simulink model "TST_CoVMD_TrqLeadCoord"  (R2016b)
settings: Solver=FixedStepDiscrete  StartTime=0.0  StopTime=simTime  FixedStep=sampleTime  RelTol=1e-3
values from neighbouring files (symbols this model uses):
  testCase = 1    [initTST_CoVMD_TrqLeadCoord_001.m]    (also in initTST_CoVMD_TrqLeadCoord_002.m = 2; initTST_CoVMD_TrqLeadCoord_003.m = 3)
libraries: simulink x16, UnitTest_Lib x12
settings Model: Creator=zhengjinyan  LastModifiedBy=zhengjinyan
settings DebuggingCC: SignalRangeChecking=error

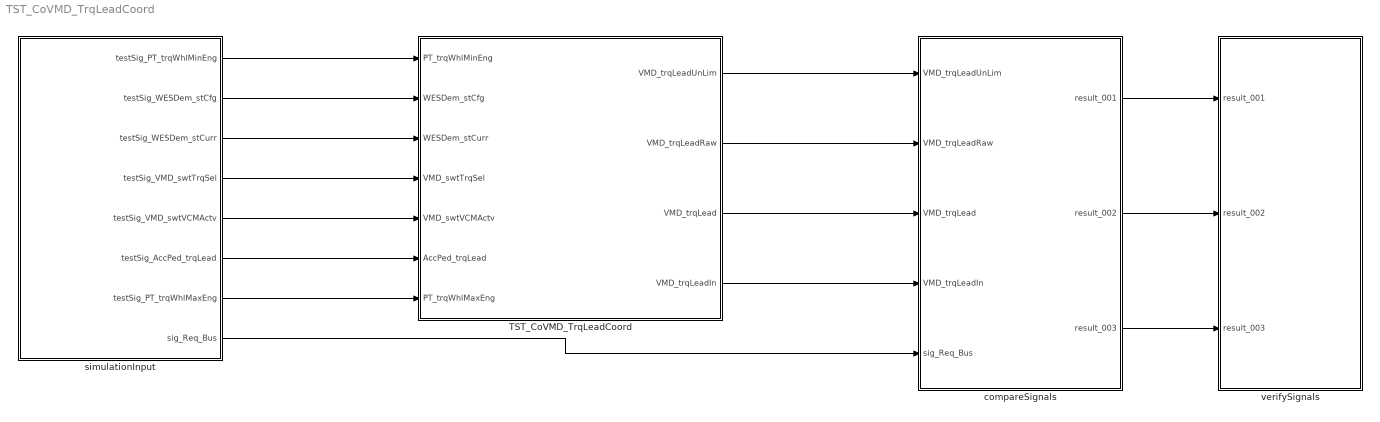
== system TST_CoVMD_TrqLeadCoord ==
  TST_CoVMD_TrqLeadCoord : Subsystem
  compareSignals : Subsystem
  simulationInput : Subsystem
  verifySignals : Subsystem
  wires:
  simulationInput/1(testSig_PT_trqWhlMinEng) -> TST_CoVMD_TrqLeadCoord/1(PT_trqWhlMinEng)
  simulationInput/2(testSig_WESDem_stCfg) -> TST_CoVMD_TrqLeadCoord/2(WESDem_stCfg)
  simulationInput/3(testSig_WESDem_stCurr) -> TST_CoVMD_TrqLeadCoord/3(WESDem_stCurr)
  simulationInput/4(testSig_VMD_swtTrqSel) -> TST_CoVMD_TrqLeadCoord/4(VMD_swtTrqSel)
  simulationInput/5(testSig_VMD_swtVCMActv) -> TST_CoVMD_TrqLeadCoord/5(VMD_swtVCMActv)
  simulationInput/6(testSig_AccPed_trqLead) -> TST_CoVMD_TrqLeadCoord/6(AccPed_trqLead)
  simulationInput/7(testSig_PT_trqWhlMaxEng) -> TST_CoVMD_TrqLeadCoord/7(PT_trqWhlMaxEng)
  TST_CoVMD_TrqLeadCoord/1(VMD_trqLeadUnLim) -> compareSignals/1(VMD_trqLeadUnLim)
  TST_CoVMD_TrqLeadCoord/2(VMD_trqLeadRaw) -> compareSignals/2(VMD_trqLeadRaw)
  TST_CoVMD_TrqLeadCoord/3(VMD_trqLead) -> compareSignals/3(VMD_trqLead)
  TST_CoVMD_TrqLeadCoord/4(VMD_trqLeadIn) -> compareSignals/4(VMD_trqLeadIn)
  simulationInput/8(sig_Req_Bus) -> compareSignals/5(sig_Req_Bus)
  compareSignals/1(result_001) -> verifySignals/1(result_001)
  compareSignals/2(result_002) -> verifySignals/2(result_002)
  compareSignals/3(result_003) -> verifySignals/3(result_003)

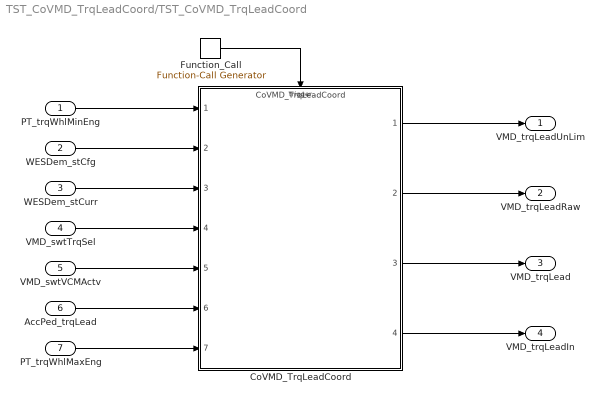
== system TST_CoVMD_TrqLeadCoord/TST_CoVMD_TrqLeadCoord ==
  PT_trqWhlMinEng : Inport
  WESDem_stCfg : Inport  Port=2
  WESDem_stCurr : Inport  Port=3
  VMD_swtTrqSel : Inport  Port=4
  VMD_swtVCMActv : Inport  Port=5
  AccPed_trqLead : Inport  Port=6
  PT_trqWhlMaxEng : Inport  Port=7
  CoVMD_TrqLeadCoord : ModelReference  ModelNameDialog=CoVMD_TrqLeadCoord  SimulationMode=Normal  ModelReferenceVersion=1.13  TriggerPortName=function  TriggerPortTriggerType=function-call  TriggerPortStatesWhenEnabling=held
  Function_Call : simulink/Ports & Subsystems/Function-Call Generator  sample_time=sampleTime  numberOfIterations=1
  VMD_trqLeadUnLim : Outport
  VMD_trqLeadRaw : Outport  Port=2
  VMD_trqLead : Outport  Port=3
  VMD_trqLeadIn : Outport  Port=4
  wires:
  Function_Call/1 -> CoVMD_TrqLeadCoord/Trigger
  PT_trqWhlMinEng/1 -> CoVMD_TrqLeadCoord/1
  WESDem_stCfg/1 -> CoVMD_TrqLeadCoord/2
  WESDem_stCurr/1 -> CoVMD_TrqLeadCoord/3
  VMD_swtTrqSel/1 -> CoVMD_TrqLeadCoord/4
  VMD_swtVCMActv/1 -> CoVMD_TrqLeadCoord/5
  AccPed_trqLead/1 -> CoVMD_TrqLeadCoord/6
  PT_trqWhlMaxEng/1 -> CoVMD_TrqLeadCoord/7
  CoVMD_TrqLeadCoord/1 -> VMD_trqLeadUnLim/1
  CoVMD_TrqLeadCoord/2 -> VMD_trqLeadRaw/1
  CoVMD_TrqLeadCoord/3 -> VMD_trqLead/1
  CoVMD_TrqLeadCoord/4 -> VMD_trqLeadIn/1

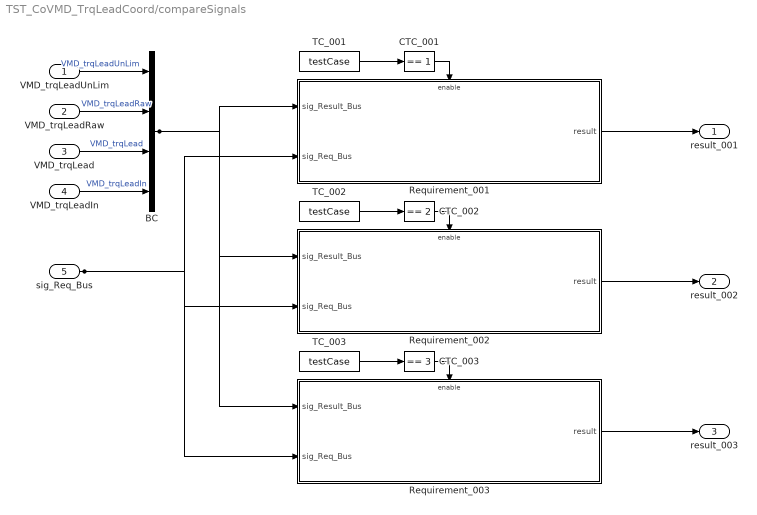
== system TST_CoVMD_TrqLeadCoord/compareSignals ==
  VMD_trqLeadUnLim : Inport
  VMD_trqLeadRaw : Inport  Port=2
  VMD_trqLead : Inport  Port=3
  VMD_trqLeadIn : Inport  Port=4
  sig_Req_Bus : Inport  Port=5
  BC : BusCreator  Inputs=4
  CTC_001 : simulink/Logic and Bit Operations/Compare To Constant  relop===  const=1  OutDataTypeStr=boolean
  CTC_002 : simulink/Logic and Bit Operations/Compare To Constant  relop===  const=2  OutDataTypeStr=boolean
  CTC_003 : simulink/Logic and Bit Operations/Compare To Constant  relop===  const=3  OutDataTypeStr=boolean
  Requirement_001 : Subsystem
  Requirement_002 : Subsystem
  Requirement_003 : Subsystem
  TC_001 : Constant  Value=testCase
  TC_002 : Constant  Value=testCase
  TC_003 : Constant  Value=testCase
  result_001 : Outport
  result_002 : Outport  Port=2
  result_003 : Outport  Port=3
  wires:
  VMD_trqLeadUnLim/1 -> BC/1  "VMD_trqLeadUnLim"
  VMD_trqLeadRaw/1 -> BC/2  "VMD_trqLeadRaw"
  VMD_trqLead/1 -> BC/3  "VMD_trqLead"
  VMD_trqLeadIn/1 -> BC/4  "VMD_trqLeadIn"
  TC_001/1 -> CTC_001/1
  CTC_001/1 -> Requirement_001/Enable
  sig_Req_Bus/1 -> Requirement_001/2(sig_Req_Bus), Requirement_002/2(sig_Req_Bus), Requirement_003/2(sig_Req_Bus)
  BC/1 -> Requirement_001/1(sig_Result_Bus), Requirement_002/1(sig_Result_Bus), Requirement_003/1(sig_Result_Bus)
  Requirement_001/1(result) -> result_001/1
  TC_002/1 -> CTC_002/1
  CTC_002/1 -> Requirement_002/Enable
  Requirement_002/1(result) -> result_002/1
  TC_003/1 -> CTC_003/1
  CTC_003/1 -> Requirement_003/Enable
  Requirement_003/1(result) -> result_003/1

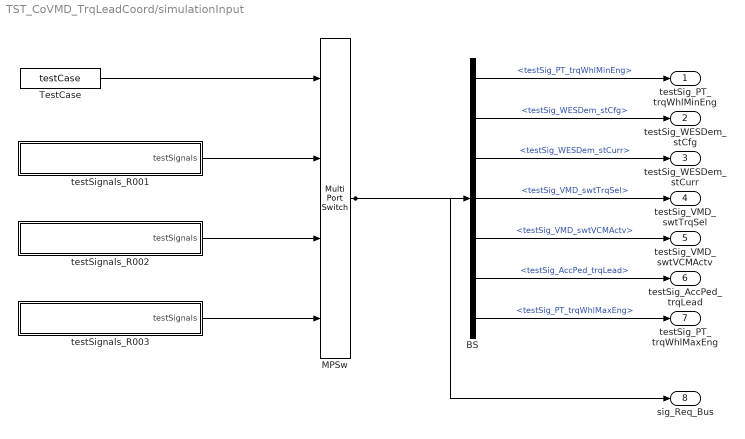
== system TST_CoVMD_TrqLeadCoord/simulationInput ==
  BS : BusSelector  OutputSignals=testSig_PT_trqWhlMinEng,testSig_WESDem_stCfg,testSig_WESDem_stCurr,testSig_VMD_swtTrqSel,testSig_VMD_swtVCMActv,testSig_AccPed_trqLead,testSig_PT_trqWhlMaxEng
  MPSw : MultiPortSwitch  SaturateOnIntegerOverflow=on  InputSameDT=on
  TestCase : Constant  Value=testCase
  testSignals_R001 : Subsystem
  testSignals_R002 : Subsystem
  testSignals_R003 : Subsystem
  testSig_PT_trqWhlMinEng : Outport
  testSig_WESDem_stCfg : Outport  Port=2
  testSig_WESDem_stCurr : Outport  Port=3
  testSig_VMD_swtTrqSel : Outport  Port=4
  testSig_VMD_swtVCMActv : Outport  Port=5
  testSig_AccPed_trqLead : Outport  Port=6
  testSig_PT_trqWhlMaxEng : Outport  Port=7
  sig_Req_Bus : Outport  Port=8
  wires:
  BS/1 -> testSig_PT_trqWhlMinEng/1  "<testSig_PT_trqWhlMinEng>"
  BS/2 -> testSig_WESDem_stCfg/1  "<testSig_WESDem_stCfg>"
  BS/3 -> testSig_WESDem_stCurr/1  "<testSig_WESDem_stCurr>"
  BS/4 -> testSig_VMD_swtTrqSel/1  "<testSig_VMD_swtTrqSel>"
  BS/5 -> testSig_VMD_swtVCMActv/1  "<testSig_VMD_swtVCMActv>"
  BS/6 -> testSig_AccPed_trqLead/1  "<testSig_AccPed_trqLead>"
  BS/7 -> testSig_PT_trqWhlMaxEng/1  "<testSig_PT_trqWhlMaxEng>"
  MPSw/1 -> BS/1, sig_Req_Bus/1
  TestCase/1 -> MPSw/1
  testSignals_R001/1(testSignals) -> MPSw/2
  testSignals_R002/1(testSignals) -> MPSw/3
  testSignals_R003/1(testSignals) -> MPSw/4

== system TST_CoVMD_TrqLeadCoord/verifySignals ==
  result_001 : Inport
  result_002 : Inport  Port=2
  result_003 : Inport  Port=3
  Assertion_001 : Assertion  Enabled=off
  Assertion_002 : Assertion  Enabled=off
  Assertion_003 : Assertion  Enabled=off
  wires:
  result_001/1 -> Assertion_001/1
  result_002/1 -> Assertion_002/1
  result_003/1 -> Assertion_003/1

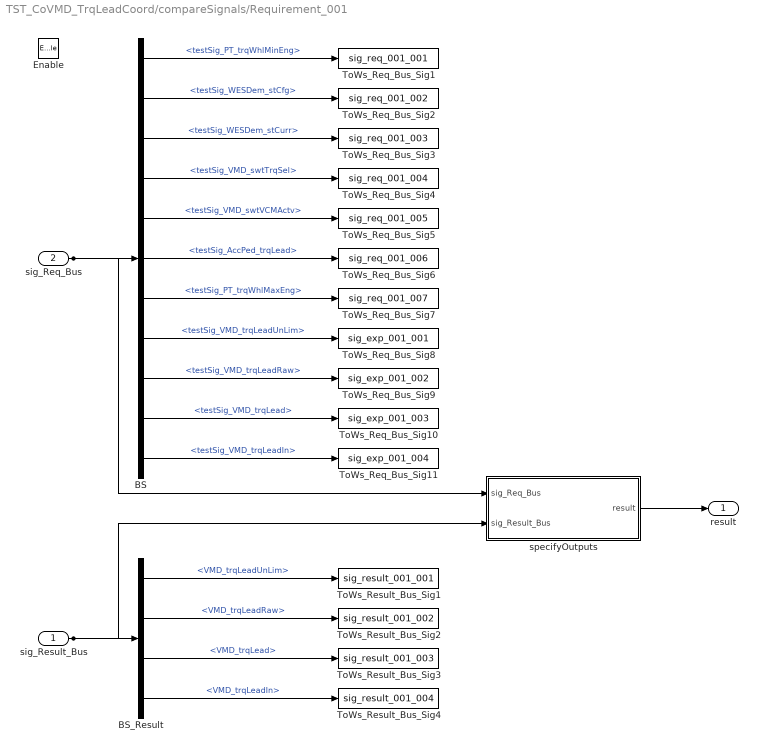
== system TST_CoVMD_TrqLeadCoord/compareSignals/Requirement_001 ==
  sig_Result_Bus : Inport
  sig_Req_Bus : Inport  Port=2
  Enable : EnablePort
  BS : BusSelector  OutputSignals=testSig_PT_trqWhlMinEng,testSig_WESDem_stCfg,testSig_WESDem_stCurr,testSig_VMD_swtTrqSel,testSig_VMD_swtVCMActv,testSig_AccPed_trqLead,testSig_PT_trqWhlMaxEng,testSig_VMD_trqLeadUnLim,testSig_VMD_trqLeadRaw,testSig_VMD_trqLead,testSig_VMD_trqLeadIn
  BS_Result : BusSelector  OutputSignals=VMD_trqLeadUnLim,VMD_trqLeadRaw,VMD_trqLead,VMD_trqLeadIn
  ToWs_Req_Bus_Sig1 : ToWorkspace  VariableName=sig_req_001_001  SaveFormat=Structure With Time
  ToWs_Req_Bus_Sig10 : ToWorkspace  VariableName=sig_exp_001_003  SaveFormat=Structure With Time
  ToWs_Req_Bus_Sig11 : ToWorkspace  VariableName=sig_exp_001_004  SaveFormat=Structure With Time
  ToWs_Req_Bus_Sig2 : ToWorkspace  VariableName=sig_req_001_002  SaveFormat=Structure With Time
  ToWs_Req_Bus_Sig3 : ToWorkspace  VariableName=sig_req_001_003  SaveFormat=Structure With Time
  ToWs_Req_Bus_Sig4 : ToWorkspace  VariableName=sig_req_001_004  SaveFormat=Structure With Time
  ToWs_Req_Bus_Sig5 : ToWorkspace  VariableName=sig_req_001_005  SaveFormat=Structure With Time
  ToWs_Req_Bus_Sig6 : ToWorkspace  VariableName=sig_req_001_006  SaveFormat=Structure With Time
  ToWs_Req_Bus_Sig7 : ToWorkspace  VariableName=sig_req_001_007  SaveFormat=Structure With Time
  ToWs_Req_Bus_Sig8 : ToWorkspace  VariableName=sig_exp_001_001  SaveFormat=Structure With Time
  ToWs_Req_Bus_Sig9 : ToWorkspace  VariableName=sig_exp_001_002  SaveFormat=Structure With Time
  ToWs_Result_Bus_Sig1 : ToWorkspace  VariableName=sig_result_001_001  SaveFormat=Structure With Time
  ToWs_Result_Bus_Sig2 : ToWorkspace  VariableName=sig_result_001_002  SaveFormat=Structure With Time
  ToWs_Result_Bus_Sig3 : ToWorkspace  VariableName=sig_result_001_003  SaveFormat=Structure With Time
  ToWs_Result_Bus_Sig4 : ToWorkspace  VariableName=sig_result_001_004  SaveFormat=Structure With Time
  specifyOutputs : Subsystem
  result : Outport
  wires:
  sig_Req_Bus/1 -> BS/1, specifyOutputs/1(sig_Req_Bus)
  BS/1 -> ToWs_Req_Bus_Sig1/1  "<testSig_PT_trqWhlMinEng>"
  BS/2 -> ToWs_Req_Bus_Sig2/1  "<testSig_WESDem_stCfg>"
  BS/3 -> ToWs_Req_Bus_Sig3/1  "<testSig_WESDem_stCurr>"
  BS/4 -> ToWs_Req_Bus_Sig4/1  "<testSig_VMD_swtTrqSel>"
  BS/5 -> ToWs_Req_Bus_Sig5/1  "<testSig_VMD_swtVCMActv>"
  BS/6 -> ToWs_Req_Bus_Sig6/1  "<testSig_AccPed_trqLead>"
  BS/7 -> ToWs_Req_Bus_Sig7/1  "<testSig_PT_trqWhlMaxEng>"
  BS/8 -> ToWs_Req_Bus_Sig8/1  "<testSig_VMD_trqLeadUnLim>"
  BS/9 -> ToWs_Req_Bus_Sig9/1  "<testSig_VMD_trqLeadRaw>"
  BS/10 -> ToWs_Req_Bus_Sig10/1  "<testSig_VMD_trqLead>"
  BS/11 -> ToWs_Req_Bus_Sig11/1  "<testSig_VMD_trqLeadIn>"
  sig_Result_Bus/1 -> BS_Result/1, specifyOutputs/2(sig_Result_Bus)
  BS_Result/1 -> ToWs_Result_Bus_Sig1/1  "<VMD_trqLeadUnLim>"
  BS_Result/2 -> ToWs_Result_Bus_Sig2/1  "<VMD_trqLeadRaw>"
  BS_Result/3 -> ToWs_Result_Bus_Sig3/1  "<VMD_trqLead>"
  BS_Result/4 -> ToWs_Result_Bus_Sig4/1  "<VMD_trqLeadIn>"
  specifyOutputs/1(result) -> result/1

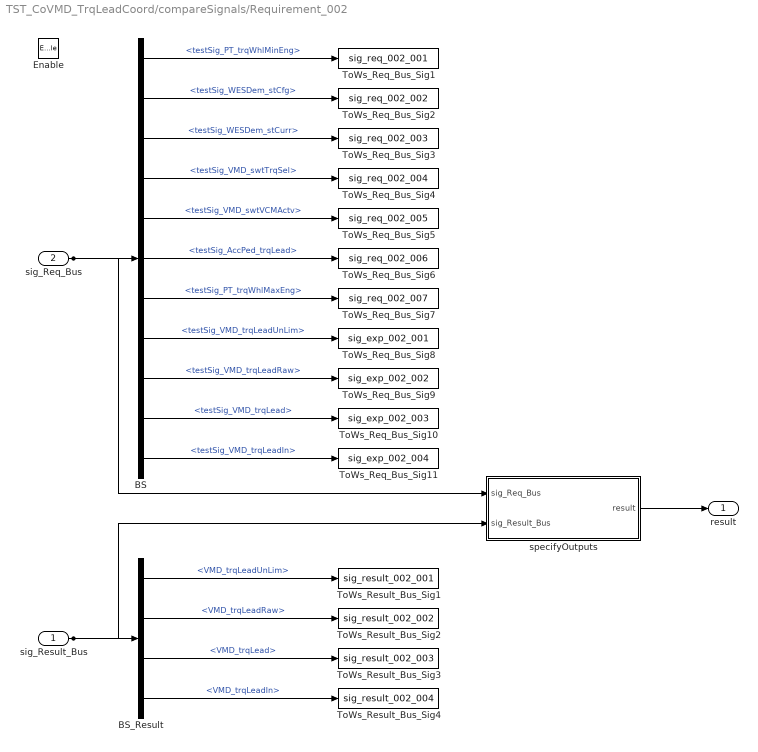
== system TST_CoVMD_TrqLeadCoord/compareSignals/Requirement_002 ==
  sig_Result_Bus : Inport
  sig_Req_Bus : Inport  Port=2
  Enable : EnablePort
  BS : BusSelector  OutputSignals=testSig_PT_trqWhlMinEng,testSig_WESDem_stCfg,testSig_WESDem_stCurr,testSig_VMD_swtTrqSel,testSig_VMD_swtVCMActv,testSig_AccPed_trqLead,testSig_PT_trqWhlMaxEng,testSig_VMD_trqLeadUnLim,testSig_VMD_trqLeadRaw,testSig_VMD_trqLead,testSig_VMD_trqLeadIn
  BS_Result : BusSelector  OutputSignals=VMD_trqLeadUnLim,VMD_trqLeadRaw,VMD_trqLead,VMD_trqLeadIn
  ToWs_Req_Bus_Sig1 : ToWorkspace  VariableName=sig_req_002_001  SaveFormat=Structure With Time
  ToWs_Req_Bus_Sig10 : ToWorkspace  VariableName=sig_exp_002_003  SaveFormat=Structure With Time
  ToWs_Req_Bus_Sig11 : ToWorkspace  VariableName=sig_exp_002_004  SaveFormat=Structure With Time
  ToWs_Req_Bus_Sig2 : ToWorkspace  VariableName=sig_req_002_002  SaveFormat=Structure With Time
  ToWs_Req_Bus_Sig3 : ToWorkspace  VariableName=sig_req_002_003  SaveFormat=Structure With Time
  ToWs_Req_Bus_Sig4 : ToWorkspace  VariableName=sig_req_002_004  SaveFormat=Structure With Time
  ToWs_Req_Bus_Sig5 : ToWorkspace  VariableName=sig_req_002_005  SaveFormat=Structure With Time
  ToWs_Req_Bus_Sig6 : ToWorkspace  VariableName=sig_req_002_006  SaveFormat=Structure With Time
  ToWs_Req_Bus_Sig7 : ToWorkspace  VariableName=sig_req_002_007  SaveFormat=Structure With Time
  ToWs_Req_Bus_Sig8 : ToWorkspace  VariableName=sig_exp_002_001  SaveFormat=Structure With Time
  ToWs_Req_Bus_Sig9 : ToWorkspace  VariableName=sig_exp_002_002  SaveFormat=Structure With Time
  ToWs_Result_Bus_Sig1 : ToWorkspace  VariableName=sig_result_002_001  SaveFormat=Structure With Time
  ToWs_Result_Bus_Sig2 : ToWorkspace  VariableName=sig_result_002_002  SaveFormat=Structure With Time
  ToWs_Result_Bus_Sig3 : ToWorkspace  VariableName=sig_result_002_003  SaveFormat=Structure With Time
  ToWs_Result_Bus_Sig4 : ToWorkspace  VariableName=sig_result_002_004  SaveFormat=Structure With Time
  specifyOutputs : Subsystem
  result : Outport
  wires:
  sig_Req_Bus/1 -> BS/1, specifyOutputs/1(sig_Req_Bus)
  BS/1 -> ToWs_Req_Bus_Sig1/1  "<testSig_PT_trqWhlMinEng>"
  BS/2 -> ToWs_Req_Bus_Sig2/1  "<testSig_WESDem_stCfg>"
  BS/3 -> ToWs_Req_Bus_Sig3/1  "<testSig_WESDem_stCurr>"
  BS/4 -> ToWs_Req_Bus_Sig4/1  "<testSig_VMD_swtTrqSel>"
  BS/5 -> ToWs_Req_Bus_Sig5/1  "<testSig_VMD_swtVCMActv>"
  BS/6 -> ToWs_Req_Bus_Sig6/1  "<testSig_AccPed_trqLead>"
  BS/7 -> ToWs_Req_Bus_Sig7/1  "<testSig_PT_trqWhlMaxEng>"
  BS/8 -> ToWs_Req_Bus_Sig8/1  "<testSig_VMD_trqLeadUnLim>"
  BS/9 -> ToWs_Req_Bus_Sig9/1  "<testSig_VMD_trqLeadRaw>"
  BS/10 -> ToWs_Req_Bus_Sig10/1  "<testSig_VMD_trqLead>"
  BS/11 -> ToWs_Req_Bus_Sig11/1  "<testSig_VMD_trqLeadIn>"
  sig_Result_Bus/1 -> BS_Result/1, specifyOutputs/2(sig_Result_Bus)
  BS_Result/1 -> ToWs_Result_Bus_Sig1/1  "<VMD_trqLeadUnLim>"
  BS_Result/2 -> ToWs_Result_Bus_Sig2/1  "<VMD_trqLeadRaw>"
  BS_Result/3 -> ToWs_Result_Bus_Sig3/1  "<VMD_trqLead>"
  BS_Result/4 -> ToWs_Result_Bus_Sig4/1  "<VMD_trqLeadIn>"
  specifyOutputs/1(result) -> result/1

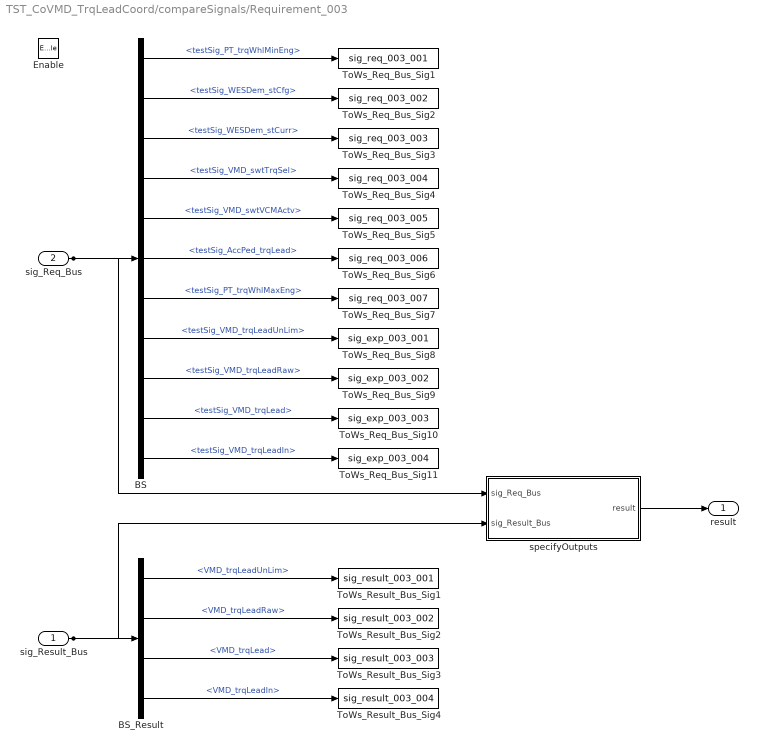
== system TST_CoVMD_TrqLeadCoord/compareSignals/Requirement_003 ==
  sig_Result_Bus : Inport
  sig_Req_Bus : Inport  Port=2
  Enable : EnablePort
  BS : BusSelector  OutputSignals=testSig_PT_trqWhlMinEng,testSig_WESDem_stCfg,testSig_WESDem_stCurr,testSig_VMD_swtTrqSel,testSig_VMD_swtVCMActv,testSig_AccPed_trqLead,testSig_PT_trqWhlMaxEng,testSig_VMD_trqLeadUnLim,testSig_VMD_trqLeadRaw,testSig_VMD_trqLead,testSig_VMD_trqLeadIn
  BS_Result : BusSelector  OutputSignals=VMD_trqLeadUnLim,VMD_trqLeadRaw,VMD_trqLead,VMD_trqLeadIn
  ToWs_Req_Bus_Sig1 : ToWorkspace  VariableName=sig_req_003_001  SaveFormat=Structure With Time
  ToWs_Req_Bus_Sig10 : ToWorkspace  VariableName=sig_exp_003_003  SaveFormat=Structure With Time
  ToWs_Req_Bus_Sig11 : ToWorkspace  VariableName=sig_exp_003_004  SaveFormat=Structure With Time
  ToWs_Req_Bus_Sig2 : ToWorkspace  VariableName=sig_req_003_002  SaveFormat=Structure With Time
  ToWs_Req_Bus_Sig3 : ToWorkspace  VariableName=sig_req_003_003  SaveFormat=Structure With Time
  ToWs_Req_Bus_Sig4 : ToWorkspace  VariableName=sig_req_003_004  SaveFormat=Structure With Time
  ToWs_Req_Bus_Sig5 : ToWorkspace  VariableName=sig_req_003_005  SaveFormat=Structure With Time
  ToWs_Req_Bus_Sig6 : ToWorkspace  VariableName=sig_req_003_006  SaveFormat=Structure With Time
  ToWs_Req_Bus_Sig7 : ToWorkspace  VariableName=sig_req_003_007  SaveFormat=Structure With Time
  ToWs_Req_Bus_Sig8 : ToWorkspace  VariableName=sig_exp_003_001  SaveFormat=Structure With Time
  ToWs_Req_Bus_Sig9 : ToWorkspace  VariableName=sig_exp_003_002  SaveFormat=Structure With Time
  ToWs_Result_Bus_Sig1 : ToWorkspace  VariableName=sig_result_003_001  SaveFormat=Structure With Time
  ToWs_Result_Bus_Sig2 : ToWorkspace  VariableName=sig_result_003_002  SaveFormat=Structure With Time
  ToWs_Result_Bus_Sig3 : ToWorkspace  VariableName=sig_result_003_003  SaveFormat=Structure With Time
  ToWs_Result_Bus_Sig4 : ToWorkspace  VariableName=sig_result_003_004  SaveFormat=Structure With Time
  specifyOutputs : Subsystem
  result : Outport
  wires:
  sig_Req_Bus/1 -> BS/1, specifyOutputs/1(sig_Req_Bus)
  BS/1 -> ToWs_Req_Bus_Sig1/1  "<testSig_PT_trqWhlMinEng>"
  BS/2 -> ToWs_Req_Bus_Sig2/1  "<testSig_WESDem_stCfg>"
  BS/3 -> ToWs_Req_Bus_Sig3/1  "<testSig_WESDem_stCurr>"
  BS/4 -> ToWs_Req_Bus_Sig4/1  "<testSig_VMD_swtTrqSel>"
  BS/5 -> ToWs_Req_Bus_Sig5/1  "<testSig_VMD_swtVCMActv>"
  BS/6 -> ToWs_Req_Bus_Sig6/1  "<testSig_AccPed_trqLead>"
  BS/7 -> ToWs_Req_Bus_Sig7/1  "<testSig_PT_trqWhlMaxEng>"
  BS/8 -> ToWs_Req_Bus_Sig8/1  "<testSig_VMD_trqLeadUnLim>"
  BS/9 -> ToWs_Req_Bus_Sig9/1  "<testSig_VMD_trqLeadRaw>"
  BS/10 -> ToWs_Req_Bus_Sig10/1  "<testSig_VMD_trqLead>"
  BS/11 -> ToWs_Req_Bus_Sig11/1  "<testSig_VMD_trqLeadIn>"
  sig_Result_Bus/1 -> BS_Result/1, specifyOutputs/2(sig_Result_Bus)
  BS_Result/1 -> ToWs_Result_Bus_Sig1/1  "<VMD_trqLeadUnLim>"
  BS_Result/2 -> ToWs_Result_Bus_Sig2/1  "<VMD_trqLeadRaw>"
  BS_Result/3 -> ToWs_Result_Bus_Sig3/1  "<VMD_trqLead>"
  BS_Result/4 -> ToWs_Result_Bus_Sig4/1  "<VMD_trqLeadIn>"
  specifyOutputs/1(result) -> result/1

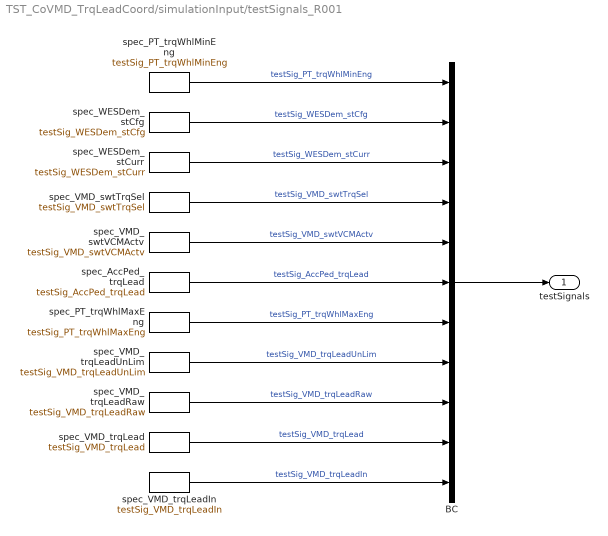
== system TST_CoVMD_TrqLeadCoord/simulationInput/testSignals_R001 ==
  BC : BusCreator  Inputs=11
  spec_AccPed_trqLead : FromWorkspace  VariableName=testSig_AccPed_trqLead  Interpolate=off  OutputAfterFinalValue=Holding final value
  spec_PT_trqWhlMaxEng : FromWorkspace  VariableName=testSig_PT_trqWhlMaxEng  Interpolate=off  OutputAfterFinalValue=Holding final value
  spec_PT_trqWhlMinEng : FromWorkspace  VariableName=testSig_PT_trqWhlMinEng  Interpolate=off  OutputAfterFinalValue=Holding final value
  spec_VMD_swtTrqSel : FromWorkspace  VariableName=testSig_VMD_swtTrqSel  Interpolate=off  OutputAfterFinalValue=Holding final value
  spec_VMD_swtVCMActv : FromWorkspace  VariableName=testSig_VMD_swtVCMActv  Interpolate=off  OutputAfterFinalValue=Holding final value
  spec_VMD_trqLead : FromWorkspace  VariableName=testSig_VMD_trqLead  Interpolate=off  OutputAfterFinalValue=Holding final value
  spec_VMD_trqLeadIn : FromWorkspace  VariableName=testSig_VMD_trqLeadIn  Interpolate=off  OutputAfterFinalValue=Holding final value
  spec_VMD_trqLeadRaw : FromWorkspace  VariableName=testSig_VMD_trqLeadRaw  Interpolate=off  OutputAfterFinalValue=Holding final value
  spec_VMD_trqLeadUnLim : FromWorkspace  VariableName=testSig_VMD_trqLeadUnLim  Interpolate=off  OutputAfterFinalValue=Holding final value
  spec_WESDem_stCfg : FromWorkspace  VariableName=testSig_WESDem_stCfg  Interpolate=off  OutputAfterFinalValue=Holding final value
  spec_WESDem_stCurr : FromWorkspace  VariableName=testSig_WESDem_stCurr  Interpolate=off  OutputAfterFinalValue=Holding final value
  testSignals : Outport
  wires:
  BC/1 -> testSignals/1
  spec_PT_trqWhlMinEng/1 -> BC/1  "testSig_PT_trqWhlMinEng"
  spec_WESDem_stCfg/1 -> BC/2  "testSig_WESDem_stCfg"
  spec_WESDem_stCurr/1 -> BC/3  "testSig_WESDem_stCurr"
  spec_VMD_swtTrqSel/1 -> BC/4  "testSig_VMD_swtTrqSel"
  spec_VMD_swtVCMActv/1 -> BC/5  "testSig_VMD_swtVCMActv"
  spec_AccPed_trqLead/1 -> BC/6  "testSig_AccPed_trqLead"
  spec_PT_trqWhlMaxEng/1 -> BC/7  "testSig_PT_trqWhlMaxEng"
  spec_VMD_trqLeadUnLim/1 -> BC/8  "testSig_VMD_trqLeadUnLim"
  spec_VMD_trqLeadRaw/1 -> BC/9  "testSig_VMD_trqLeadRaw"
  spec_VMD_trqLead/1 -> BC/10  "testSig_VMD_trqLead"
  spec_VMD_trqLeadIn/1 -> BC/11  "testSig_VMD_trqLeadIn"

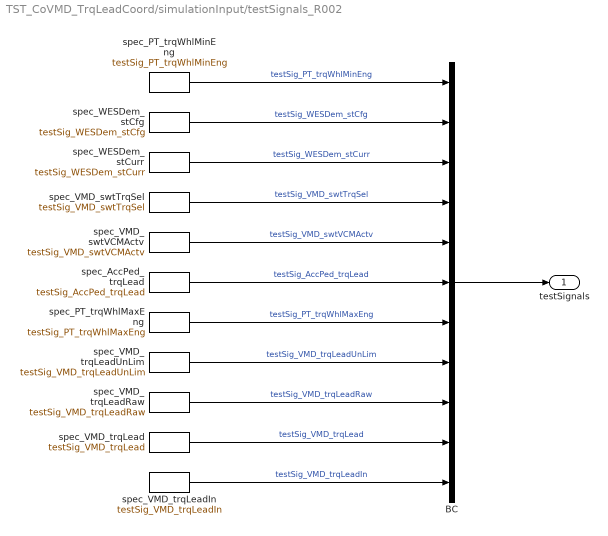
== system TST_CoVMD_TrqLeadCoord/simulationInput/testSignals_R002 ==
  BC : BusCreator  Inputs=11
  spec_AccPed_trqLead : FromWorkspace  VariableName=testSig_AccPed_trqLead  Interpolate=off  OutputAfterFinalValue=Holding final value
  spec_PT_trqWhlMaxEng : FromWorkspace  VariableName=testSig_PT_trqWhlMaxEng  Interpolate=off  OutputAfterFinalValue=Holding final value
  spec_PT_trqWhlMinEng : FromWorkspace  VariableName=testSig_PT_trqWhlMinEng  Interpolate=off  OutputAfterFinalValue=Holding final value
  spec_VMD_swtTrqSel : FromWorkspace  VariableName=testSig_VMD_swtTrqSel  Interpolate=off  OutputAfterFinalValue=Holding final value
  spec_VMD_swtVCMActv : FromWorkspace  VariableName=testSig_VMD_swtVCMActv  Interpolate=off  OutputAfterFinalValue=Holding final value
  spec_VMD_trqLead : FromWorkspace  VariableName=testSig_VMD_trqLead  Interpolate=off  OutputAfterFinalValue=Holding final value
  spec_VMD_trqLeadIn : FromWorkspace  VariableName=testSig_VMD_trqLeadIn  Interpolate=off  OutputAfterFinalValue=Holding final value
  spec_VMD_trqLeadRaw : FromWorkspace  VariableName=testSig_VMD_trqLeadRaw  Interpolate=off  OutputAfterFinalValue=Holding final value
  spec_VMD_trqLeadUnLim : FromWorkspace  VariableName=testSig_VMD_trqLeadUnLim  Interpolate=off  OutputAfterFinalValue=Holding final value
  spec_WESDem_stCfg : FromWorkspace  VariableName=testSig_WESDem_stCfg  Interpolate=off  OutputAfterFinalValue=Holding final value
  spec_WESDem_stCurr : FromWorkspace  VariableName=testSig_WESDem_stCurr  Interpolate=off  OutputAfterFinalValue=Holding final value
  testSignals : Outport
  wires:
  BC/1 -> testSignals/1
  spec_PT_trqWhlMinEng/1 -> BC/1  "testSig_PT_trqWhlMinEng"
  spec_WESDem_stCfg/1 -> BC/2  "testSig_WESDem_stCfg"
  spec_WESDem_stCurr/1 -> BC/3  "testSig_WESDem_stCurr"
  spec_VMD_swtTrqSel/1 -> BC/4  "testSig_VMD_swtTrqSel"
  spec_VMD_swtVCMActv/1 -> BC/5  "testSig_VMD_swtVCMActv"
  spec_AccPed_trqLead/1 -> BC/6  "testSig_AccPed_trqLead"
  spec_PT_trqWhlMaxEng/1 -> BC/7  "testSig_PT_trqWhlMaxEng"
  spec_VMD_trqLeadUnLim/1 -> BC/8  "testSig_VMD_trqLeadUnLim"
  spec_VMD_trqLeadRaw/1 -> BC/9  "testSig_VMD_trqLeadRaw"
  spec_VMD_trqLead/1 -> BC/10  "testSig_VMD_trqLead"
  spec_VMD_trqLeadIn/1 -> BC/11  "testSig_VMD_trqLeadIn"

== system TST_CoVMD_TrqLeadCoord/simulationInput/testSignals_R003 ==
  BC : BusCreator  Inputs=11
  spec_AccPed_trqLead : FromWorkspace  VariableName=testSig_AccPed_trqLead  Interpolate=off  OutputAfterFinalValue=Holding final value
  spec_PT_trqWhlMaxEng : FromWorkspace  VariableName=testSig_PT_trqWhlMaxEng  Interpolate=off  OutputAfterFinalValue=Holding final value
  spec_PT_trqWhlMinEng : FromWorkspace  VariableName=testSig_PT_trqWhlMinEng  Interpolate=off  OutputAfterFinalValue=Holding final value
  spec_VMD_swtTrqSel : FromWorkspace  VariableName=testSig_VMD_swtTrqSel  Interpolate=off  OutputAfterFinalValue=Holding final value
  spec_VMD_swtVCMActv : FromWorkspace  VariableName=testSig_VMD_swtVCMActv  Interpolate=off  OutputAfterFinalValue=Holding final value
  spec_VMD_trqLead : FromWorkspace  VariableName=testSig_VMD_trqLead  Interpolate=off  OutputAfterFinalValue=Holding final value
  spec_VMD_trqLeadIn : FromWorkspace  VariableName=testSig_VMD_trqLeadIn  Interpolate=off  OutputAfterFinalValue=Holding final value
  spec_VMD_trqLeadRaw : FromWorkspace  VariableName=testSig_VMD_trqLeadRaw  Interpolate=off  OutputAfterFinalValue=Holding final value
  spec_VMD_trqLeadUnLim : FromWorkspace  VariableName=testSig_VMD_trqLeadUnLim  Interpolate=off  OutputAfterFinalValue=Holding final value
  spec_WESDem_stCfg : FromWorkspace  VariableName=testSig_WESDem_stCfg  Interpolate=off  OutputAfterFinalValue=Holding final value
  spec_WESDem_stCurr : FromWorkspace  VariableName=testSig_WESDem_stCurr  Interpolate=off  OutputAfterFinalValue=Holding final value
  testSignals : Outport
  wires:
  BC/1 -> testSignals/1
  spec_PT_trqWhlMinEng/1 -> BC/1  "testSig_PT_trqWhlMinEng"
  spec_WESDem_stCfg/1 -> BC/2  "testSig_WESDem_stCfg"
  spec_WESDem_stCurr/1 -> BC/3  "testSig_WESDem_stCurr"
  spec_VMD_swtTrqSel/1 -> BC/4  "testSig_VMD_swtTrqSel"
  spec_VMD_swtVCMActv/1 -> BC/5  "testSig_VMD_swtVCMActv"
  spec_AccPed_trqLead/1 -> BC/6  "testSig_AccPed_trqLead"
  spec_PT_trqWhlMaxEng/1 -> BC/7  "testSig_PT_trqWhlMaxEng"
  spec_VMD_trqLeadUnLim/1 -> BC/8  "testSig_VMD_trqLeadUnLim"
  spec_VMD_trqLeadRaw/1 -> BC/9  "testSig_VMD_trqLeadRaw"
  spec_VMD_trqLead/1 -> BC/10  "testSig_VMD_trqLead"
  spec_VMD_trqLeadIn/1 -> BC/11  "testSig_VMD_trqLeadIn"

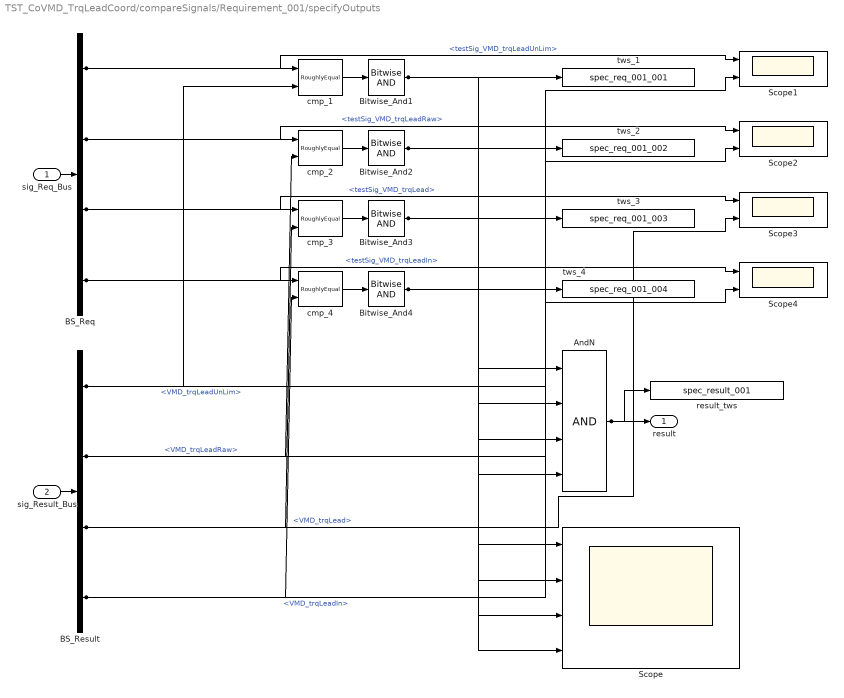
== system TST_CoVMD_TrqLeadCoord/compareSignals/Requirement_001/specifyOutputs ==
  sig_Req_Bus : Inport
  sig_Result_Bus : Inport  Port=2
  AndN : Logic  Inputs=4
  BS_Req : BusSelector  OutputSignals=testSig_VMD_trqLeadUnLim,testSig_VMD_trqLeadRaw,testSig_VMD_trqLead,testSig_VMD_trqLeadIn
  BS_Result : BusSelector  OutputSignals=VMD_trqLeadUnLim,VMD_trqLeadRaw,VMD_trqLead,VMD_trqLeadIn
  Bitwise_And{1..4} (4 alike) : simulink/Logic and Bit Operations/Bitwise Operator  logicop=AND  UseBitMask=off  BitMask=bin2dec('11011001')  BitMaskRealWorld=Stored Integer
  Scope : Scope  NumInputPorts=4
  Scope{1..4} (4 alike) : Scope  NumInputPorts=2
  cmp_{1..4} (4 alike) : UnitTest_Lib/RoughlyEqual  slope=0.1
  result_tws : ToWorkspace  VariableName=spec_result_001
  tws_1 : ToWorkspace  VariableName=spec_req_001_001
  tws_2 : ToWorkspace  VariableName=spec_req_001_002
  tws_3 : ToWorkspace  VariableName=spec_req_001_003
  tws_4 : ToWorkspace  VariableName=spec_req_001_004
  result : Outport
  wires:
  sig_Req_Bus/1 -> BS_Req/1
  sig_Result_Bus/1 -> BS_Result/1
  AndN/1 -> result/1, result_tws/1
  BS_Req/1 -> cmp_1/1, Scope1/1  "<testSig_VMD_trqLeadUnLim>"
  BS_Result/1 -> cmp_1/2, Scope1/2  "<VMD_trqLeadUnLim>"
  cmp_1/1 -> Bitwise_And1/1
  Bitwise_And1/1 -> tws_1/1, AndN/1, Scope/1
  BS_Req/2 -> cmp_2/1, Scope2/1  "<testSig_VMD_trqLeadRaw>"
  BS_Result/2 -> cmp_2/2, Scope2/2  "<VMD_trqLeadRaw>"
  cmp_2/1 -> Bitwise_And2/1
  Bitwise_And2/1 -> tws_2/1, AndN/2, Scope/2
  BS_Req/3 -> cmp_3/1, Scope3/1  "<testSig_VMD_trqLead>"
  BS_Result/3 -> cmp_3/2, Scope3/2  "<VMD_trqLead>"
  cmp_3/1 -> Bitwise_And3/1
  Bitwise_And3/1 -> tws_3/1, AndN/3, Scope/3
  BS_Req/4 -> cmp_4/1, Scope4/1  "<testSig_VMD_trqLeadIn>"
  BS_Result/4 -> cmp_4/2, Scope4/2  "<VMD_trqLeadIn>"
  cmp_4/1 -> Bitwise_And4/1
  Bitwise_And4/1 -> tws_4/1, AndN/4, Scope/4

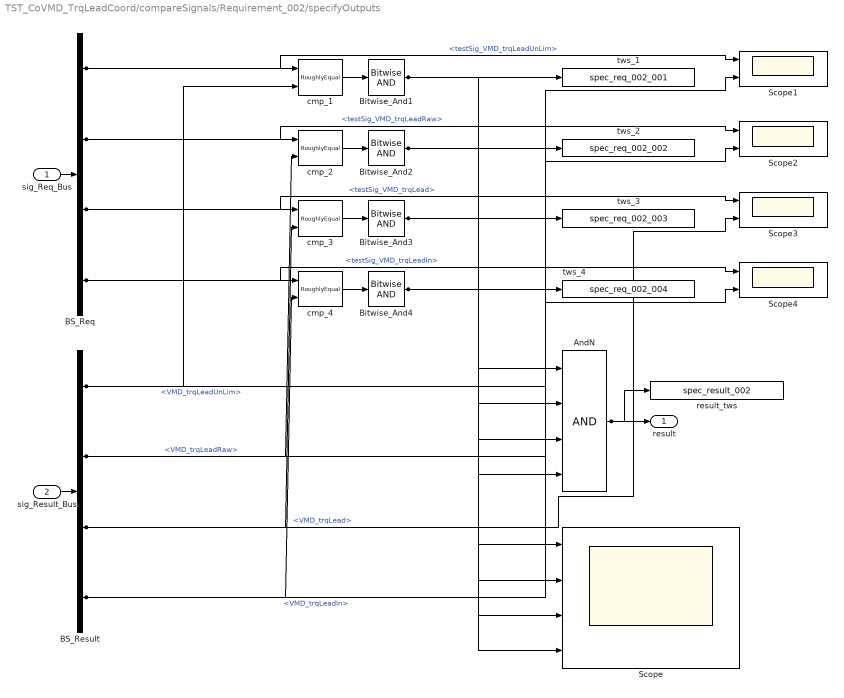
== system TST_CoVMD_TrqLeadCoord/compareSignals/Requirement_002/specifyOutputs ==
  sig_Req_Bus : Inport
  sig_Result_Bus : Inport  Port=2
  AndN : Logic  Inputs=4
  BS_Req : BusSelector  OutputSignals=testSig_VMD_trqLeadUnLim,testSig_VMD_trqLeadRaw,testSig_VMD_trqLead,testSig_VMD_trqLeadIn
  BS_Result : BusSelector  OutputSignals=VMD_trqLeadUnLim,VMD_trqLeadRaw,VMD_trqLead,VMD_trqLeadIn
  Bitwise_And{1..4} (4 alike) : simulink/Logic and Bit Operations/Bitwise Operator  logicop=AND  UseBitMask=off  BitMask=bin2dec('11011001')  BitMaskRealWorld=Stored Integer
  Scope : Scope  NumInputPorts=4
  Scope{1..4} (4 alike) : Scope  NumInputPorts=2
  cmp_{1..4} (4 alike) : UnitTest_Lib/RoughlyEqual  slope=0.1
  result_tws : ToWorkspace  VariableName=spec_result_002
  tws_1 : ToWorkspace  VariableName=spec_req_002_001
  tws_2 : ToWorkspace  VariableName=spec_req_002_002
  tws_3 : ToWorkspace  VariableName=spec_req_002_003
  tws_4 : ToWorkspace  VariableName=spec_req_002_004
  result : Outport
  wires:
  sig_Req_Bus/1 -> BS_Req/1
  sig_Result_Bus/1 -> BS_Result/1
  AndN/1 -> result/1, result_tws/1
  BS_Req/1 -> cmp_1/1, Scope1/1  "<testSig_VMD_trqLeadUnLim>"
  BS_Result/1 -> cmp_1/2, Scope1/2  "<VMD_trqLeadUnLim>"
  cmp_1/1 -> Bitwise_And1/1
  Bitwise_And1/1 -> tws_1/1, AndN/1, Scope/1
  BS_Req/2 -> cmp_2/1, Scope2/1  "<testSig_VMD_trqLeadRaw>"
  BS_Result/2 -> cmp_2/2, Scope2/2  "<VMD_trqLeadRaw>"
  cmp_2/1 -> Bitwise_And2/1
  Bitwise_And2/1 -> tws_2/1, AndN/2, Scope/2
  BS_Req/3 -> cmp_3/1, Scope3/1  "<testSig_VMD_trqLead>"
  BS_Result/3 -> cmp_3/2, Scope3/2  "<VMD_trqLead>"
  cmp_3/1 -> Bitwise_And3/1
  Bitwise_And3/1 -> tws_3/1, AndN/3, Scope/3
  BS_Req/4 -> cmp_4/1, Scope4/1  "<testSig_VMD_trqLeadIn>"
  BS_Result/4 -> cmp_4/2, Scope4/2  "<VMD_trqLeadIn>"
  cmp_4/1 -> Bitwise_And4/1
  Bitwise_And4/1 -> tws_4/1, AndN/4, Scope/4

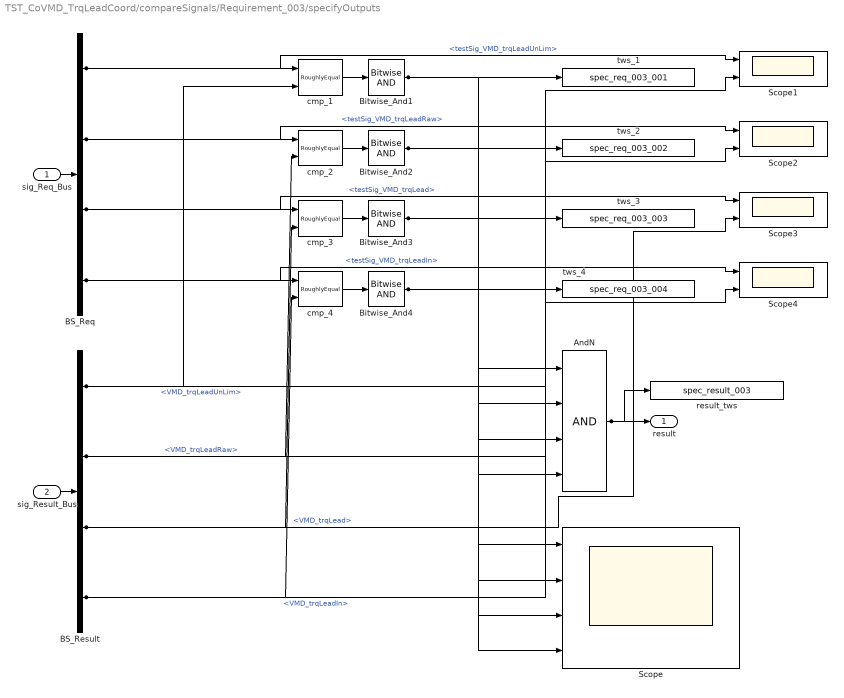
== system TST_CoVMD_TrqLeadCoord/compareSignals/Requirement_003/specifyOutputs ==
  sig_Req_Bus : Inport
  sig_Result_Bus : Inport  Port=2
  AndN : Logic  Inputs=4
  BS_Req : BusSelector  OutputSignals=testSig_VMD_trqLeadUnLim,testSig_VMD_trqLeadRaw,testSig_VMD_trqLead,testSig_VMD_trqLeadIn
  BS_Result : BusSelector  OutputSignals=VMD_trqLeadUnLim,VMD_trqLeadRaw,VMD_trqLead,VMD_trqLeadIn
  Bitwise_And{1..4} (4 alike) : simulink/Logic and Bit Operations/Bitwise Operator  logicop=AND  UseBitMask=off  BitMask=bin2dec('11011001')  BitMaskRealWorld=Stored Integer
  Scope : Scope  NumInputPorts=4
  Scope{1..4} (4 alike) : Scope  NumInputPorts=2
  cmp_{1..4} (4 alike) : UnitTest_Lib/RoughlyEqual  slope=0.1
  result_tws : ToWorkspace  VariableName=spec_result_003
  tws_1 : ToWorkspace  VariableName=spec_req_003_001
  tws_2 : ToWorkspace  VariableName=spec_req_003_002
  tws_3 : ToWorkspace  VariableName=spec_req_003_003
  tws_4 : ToWorkspace  VariableName=spec_req_003_004
  result : Outport
  wires:
  sig_Req_Bus/1 -> BS_Req/1
  sig_Result_Bus/1 -> BS_Result/1
  AndN/1 -> result/1, result_tws/1
  BS_Req/1 -> cmp_1/1, Scope1/1  "<testSig_VMD_trqLeadUnLim>"
  BS_Result/1 -> cmp_1/2, Scope1/2  "<VMD_trqLeadUnLim>"
  cmp_1/1 -> Bitwise_And1/1
  Bitwise_And1/1 -> tws_1/1, AndN/1, Scope/1
  BS_Req/2 -> cmp_2/1, Scope2/1  "<testSig_VMD_trqLeadRaw>"
  BS_Result/2 -> cmp_2/2, Scope2/2  "<VMD_trqLeadRaw>"
  cmp_2/1 -> Bitwise_And2/1
  Bitwise_And2/1 -> tws_2/1, AndN/2, Scope/2
  BS_Req/3 -> cmp_3/1, Scope3/1  "<testSig_VMD_trqLead>"
  BS_Result/3 -> cmp_3/2, Scope3/2  "<VMD_trqLead>"
  cmp_3/1 -> Bitwise_And3/1
  Bitwise_And3/1 -> tws_3/1, AndN/3, Scope/3
  BS_Req/4 -> cmp_4/1, Scope4/1  "<testSig_VMD_trqLeadIn>"
  BS_Result/4 -> cmp_4/2, Scope4/2  "<VMD_trqLeadIn>"
  cmp_4/1 -> Bitwise_And4/1
  Bitwise_And4/1 -> tws_4/1, AndN/4, Scope/4
